simulink model "model"  (R2023b)
settings: Solver=FixedStepAuto  StartTime=0.0  StopTime=500  FixedStep=T  RelTol=1e-3
undefined symbols (not defined in the file or in its folder): G_d, T, xi_0
settings Model: Creator=Denis  LastModifiedBy=Denis

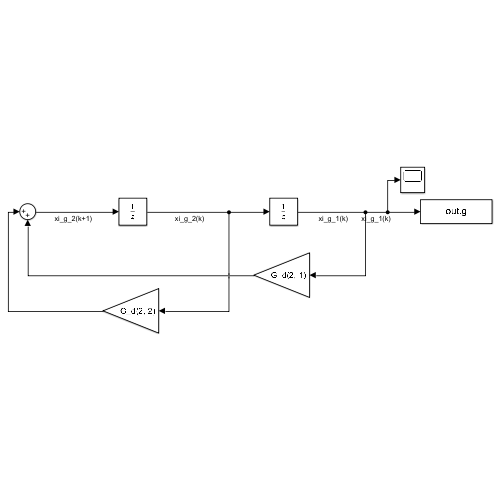
[thumbnail: Simulink's stored preview of the top-level diagram]
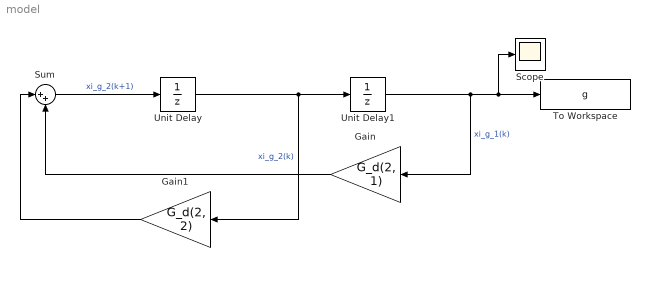
== system model ==
  Gain : Gain  Gain=G_d(2, 1)
  Gain1 : Gain  Gain=G_d(2, 2)
  Scope : Scope
  Sum : Sum  Inputs=|++
  To Workspace : ToWorkspace  VariableName=g  SaveFormat=Timeseries  SampleTime=-1
  Unit Delay : UnitDelay  InitialCondition=xi_0(2)  SampleTime=T  HasFrameUpgradeWarning=on
  Unit Delay1 : UnitDelay  InitialCondition=xi_0(1)  SampleTime=T  HasFrameUpgradeWarning=on
  wires:
  Unit Delay1/1 -> Scope/1, To Workspace/1, Gain/1  "xi_g_1(k)"
  Unit Delay/1 -> Unit Delay1/1, Gain1/1  "xi_g_2(k)"
  Sum/1 -> Unit Delay/1  "xi_g_2(k+1)"
  Gain/1 -> Sum/2
  Gain1/1 -> Sum/1
